simulink model "uni_pursuit"  (R2017a)
settings: Solver=ode45  StartTime=0.0  StopTime=104  RelTol=1e-3  EnableMultiTasking=on
StopFcn:
  | q = out.find('y');
  | figure(1), clf;
  | plot(q(:,1), q(:,2));
  | axis equal;
  | grid on;
  | 
  | goal = q(:,5:6);
  | 
  | hold on;
  | plot(robotpath(:,1), robotpath(:,2), 'r--', 'LineWidth', 2)
  | 
  | figure(2), clf;
  | mplot(out.find('t'), q,'label',{'x','y','\theta','\omega', 'x_p', 'y_p', 'v'});
  | 
  | set(0,'ShowHiddenHandles', 'on')
  | hold on
  | plot(robotpath(:,1), robotpath(:,2), 'r--', 'LineWidth', 2)
  | set(0,'ShowHiddenHandles', 'off')
values from neighbouring files (symbols this model uses):
  robotpath = my_mstraj(waypoints, vel, Ts)    [se2_motion_planning.m]
  tseg = numrows(robotpath)*Ts    [se2_motion_planning.m]
undefined symbols (not defined in the file or in its folder): numrows
libraries: simulink x1, roblocks x1, simulink_need_slupdate x1
settings Model: Creator=pic  LastModifiedBy=plusk01
settings DataIOCC: LimitDataPoints=on  MaxDataPoints=10000  SaveFormat=Array  SignalLoggingSaveFormat=ModelDataLogs  SignalLogging=off  DSMLogging=off  VisualizeSimOutput=off  ReturnWorkspaceOutputs=on  TimeSaveName=t  OutputSaveName=y
settings OptimizationCC: ExpressionDepthLimit=2147483647  LifeSpan=inf
settings DebuggingCC: UnderspecifiedInitializationDetection=Classic  MergeDetectMultiDrivingBlocksExec=none  SolverPrmCheckMsg=warning  FcnCallInpInsideContextMsg=warning  AllowSymbolicDim=off  StateNameClashWarn=warning  SFUnexpectedBacktrackingDiag=warning  SFNoUnconditionalDefaultTransitionDiag=warning  SFExecutionAtInitializationDiag=none
settings HardwareCC: ProdBitPerPointer=32  ProdBitPerSizeT=32  ProdBitPerPtrDiffT=32  ProdLargestAtomicFloat=None  ProdIntDivRoundTo=Undefined  ProdEndianess=Unspecified  ProdWordSize=32  ProdHWDeviceType=32-bit Generic
settings ModelReferenceCC: PropagateSignalLabelsOutOfModel=off
settings GRTTargetCC: TargetLangStandard=C89/C90 (ANSI)  GeneratePreprocessorConditionals=Disable all  CombineOutputUpdateFcns=off  GRTInterface=on
settings ConfigComp: CovMetricSettings=dw  CovHtmlReporting=on  CovSaveCumulativeToWorkspaceVar=on  CovSaveSingleToWorkspaceVar=on  CovExternalEMLEnable=off

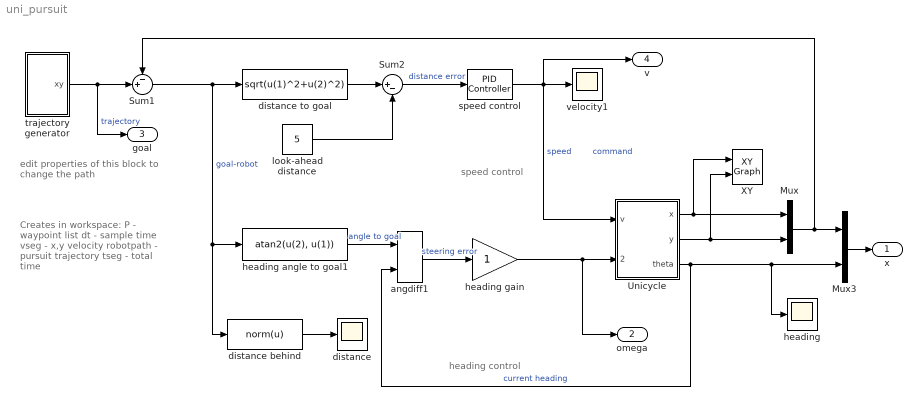
== system uni_pursuit ==
  note: edit properties
      | of this block to
      | change the path
  note: Creates in workspace:
      | P - waypoint list
      | dt - sample time
      | vseg - x,y velocity
      | robotpath - pursuit trajectory
      | tseg - total time
  note: speed control
  note: heading control
  Mux : Mux  Inputs=2
  Mux3 : Mux  Inputs=2
  Sum1 : Sum  Inputs=-+|
  Sum2 : Sum  Inputs=|+-
  Unicycle : Subsystem  mask{accel=5, vlim=5, alim=2, L=0, x0=[0, 0, 0], a=0}
      mask prompts: accel "Acceleration"; vlim "Velocity limit"; alim "Steering limits"; L "Wheel base"; x0 "Initial state (x, y, theta)"; a "Coordinate frame shift (a)"
      mask help: Kino-dynamic model of bicycle vehicle
      mask Help:
      | Kino-dynamic model of bicycle vehicle, also known as Ackermann vehicle
      | model.
      | 
      | <b>Parameters::</b>
      | 
      | Acceleration (1x1)   Vehicle acceleration limit [m/s2]
      | Velocity limit (1x1)  Vehicle speed limit [m/s]
      | Steering limits (1x1) Steering angle limit [rad]
      | Initial state (1x3) Initial state (x, y, theta)
      | Handbrake (1x1) Vehicle cannot move if non-zero
      | 
      | <b>Inputs::</b>
      | 
      | v (1x1) velocity demand [m/s]
      | gamma (1x1) steering angle [rad]
      | 
      | <b>Outputs::</b>
      | 
      | x (1x1) x-coordinate in world frame [m]
      | y (1x1) x-coordinate in world frame [m]
      | theta (1x1) heading angle in world frame [rad]
      | 
      | 
      | <b>Notes::</b>
      | 
      | - Steering limit is symmetric between -limit and +limit
      | - Same dynamic model as the Toolbox class Vehicle.
      mask Display:
      | port_label('input', 1, 'v')
      | port_label('input', 2, '\omega', 'texmode', 'on')
      | port_label('output', 1, 'x')
      | port_label('output', 2, 'y')
      | port_label('output', 3, '\theta', 'texmode', 'on')
  XY : simulink/Sinks/XY Graph  xmin=0  xmax=100  ymin=0  ymax=100  st=-1
  angdiff1 : roblocks/Toolbox/angdiff
  distance : Scope
  distance behind : MATLABFcn  MATLABFcn=norm(u)
  distance to goal : Fcn  Expr=sqrt(u(1)^2+u(2)^2)
  heading : Scope
  heading angle to goal1 : Fcn  Expr=atan2(u(2), u(1))
  heading gain : Gain
  look-ahead distance : Constant  Value=5
  speed control : simulink_need_slupdate/PID Controller  P=0.5  I=0.1  D=0
      settings: SourceProductName=Simulink
  trajectory generator : Subsystem  InitFcn=|
      | % create a path for the robot to follow
      | 
      | waypoints =[ 
      |   10 10
      |   10 60
      |   80 80
      |   50 10
      |   40 80
      | ];
      | vseg = [2.5 2.5];
      | dt = 0.1;
      | robotpath = mstraj(waypoints(2:end,:), vseg, [], waypoints(1,:), dt, 0);
      | tseg = numrows(robotpath)*dt;
      | set_param('uni_pursuit', 'StopTime', num2str(sum(tseg)))
  velocity1 : Scope
  x : Outport
  omega : Outport  Port=2
  goal : Outport  Port=3
  v : Outport  Port=4
  wires:
  Mux3/1 -> x/1
  Unicycle/2(y) -> Mux/2, XY/2
  Unicycle/1(x) -> Mux/1, XY/1
  Mux/1 -> Sum1/1, Mux3/1
  distance behind/1 -> distance/1
  speed control/1 -> Unicycle/1(v), velocity1/1, v/1  "speed        command"
  angdiff1/1 -> heading gain/1  "steering error"
  Unicycle/3(theta) -> angdiff1/2, heading/1, Mux3/2  "current heading"
  heading angle to goal1/1 -> angdiff1/1  "angle to goal"
  Sum1/1 -> distance behind/1, heading angle to goal1/1, distance to goal/1  "goal-robot"
  heading gain/1 -> Unicycle/2(omega), omega/1
  trajectory generator/1(xy) -> goal/1, Sum1/2  "trajectory"
  Sum2/1 -> speed control/1  "distance error"
  look-ahead distance/1 -> Sum2/2
  distance to goal/1 -> Sum2/1

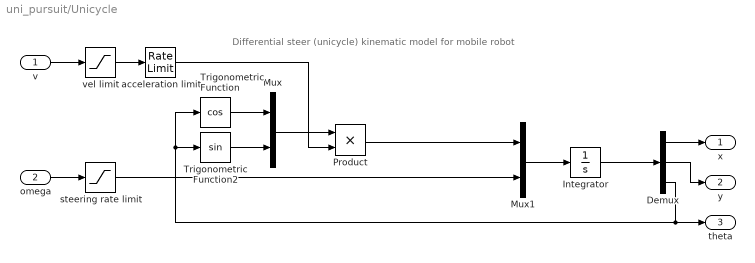
== system uni_pursuit/Unicycle ==
  note: Differential steer (unicycle) kinematic model for mobile robot
  v : Inport
  omega : Inport  Port=2
  Demux : Demux  Outputs=3
  Integrator : Integrator
  Mux : Mux  Inputs=2
  Mux1 : Mux  Inputs=2
  Product : Product  RndMeth=Zero
  Trigonometric Function : Trigonometry  Operator=cos
  Trigonometric Function2 : Trigonometry
  acceleration limit : RateLimiter  RisingSlewLimit=accel  FallingSlewLimit=-accel  SampleTimeMode=inherited
  steering rate limit : Saturate  UpperLimit=alim  LowerLimit=-alim
  vel limit : Saturate  UpperLimit=vlim  LowerLimit=-vlim
  x : Outport
  y : Outport  Port=2
  theta : Outport  Port=3
  wires:
  Trigonometric Function/1 -> Mux/1
  acceleration limit/1 -> Product/2
  Integrator/1 -> Demux/1
  Demux/3 -> Trigonometric Function/1, Trigonometric Function2/1, theta/1
  Demux/1 -> x/1
  Demux/2 -> y/1
  omega/1 -> steering rate limit/1
  v/1 -> vel limit/1
  Mux/1 -> Product/1
  vel limit/1 -> acceleration limit/1
  Trigonometric Function2/1 -> Mux/2
  steering rate limit/1 -> Mux1/2
  Mux1/1 -> Integrator/1
  Product/1 -> Mux1/1

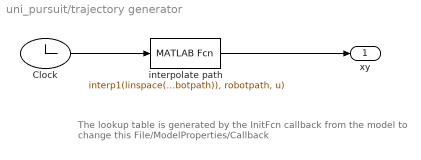
== system uni_pursuit/trajectory generator ==
  note: The lookup table is generated by the InitFcn callback from the model
      | to change this File/ModelProperties/Callback
  Clock : Clock
  interpolate path : MATLABFcn  MATLABFcn=interp1(linspace(0,tseg,numrows(robotpath)), robotpath, u)
  xy : Outport
  wires:
  Clock/1 -> interpolate path/1
  interpolate path/1 -> xy/1
